simulink model "Model"  (R2024b)
settings: Solver=VariableStepAuto  StartTime=0.0  StopTime=30  MaxStep=0.001  RelTol=1e-4
PostLoadFcn:
  | SIM_setup
values from neighbouring files (symbols this model uses):
  A = 1.1    [RT14e_Parameters.m]    (also in RT15e_Parameters.m = 1.088; RT15evo_Parameters.m = 1.088; SIM_setup.m = 1.12)
  Aero_balance = 55    [RT14e_Parameters.m]    (also in RT15e_Parameters.m; RT15evo_Parameters.m; SIM_setup.m = 0.55)
  air_density = 1.29    [SIM_setup.m]
  Br_coef_of_friction_F = 0.33    [RT14e_Parameters.m]    (also in RT15e_Parameters.m; RT15evo_Parameters.m; SIM_setup.m = 0.25)
  Br_coef_of_friction_R = 0.33    [RT14e_Parameters.m]    (also in RT15e_Parameters.m; RT15evo_Parameters.m; SIM_setup.m = 0.25)
  Br_pistons_area_F = 3617.26/1e6    (= 0.00361726)    [RT14e_Parameters.m]    (also in RT15e_Parameters.m; RT15evo_Parameters.m; SIM_setup.m)
  Br_pistons_area_R = 2026.83/1e6    (= 0.00202683)    [RT14e_Parameters.m]    (also in RT15e_Parameters.m; RT15evo_Parameters.m; SIM_setup.m)
  Cd = 1.387    [SIM_setup.m]
  Cl = 3.299    [SIM_setup.m]
  CoG_z = 0.35    [RT14e_Parameters.m]    (also in RT15e_Parameters.m = 0.28495; RT15evo_Parameters.m = 0.28495; SIM_setup.m = 0.328)
  Default_Fz_F = g*(Mass*(Lr/Wheelbase))    [RT14e_Parameters.m]    (also in RT15e_Parameters.m; RT15evo_Parameters.m; SIM_setup.m = 608.22)
  Default_Fz_R = g*(Mass*(Lf/Wheelbase))    [RT14e_Parameters.m]    (also in RT15e_Parameters.m; RT15evo_Parameters.m; SIM_setup.m = 774.99)
  Effective_br_disk_r_F = 0.0905    [RT14e_Parameters.m]    (also in RT15e_Parameters.m; RT15evo_Parameters.m; SIM_setup.m)
  Effective_br_disk_r_R = 0.0895    [RT14e_Parameters.m]    (also in RT15e_Parameters.m; RT15evo_Parameters.m; SIM_setup.m)
  Fx = Data_Fx(2:end,3:end)    [RT14e_Parameters.m]    (also in RT15e_Parameters.m; RT15evo_Parameters.m; SIM_setup.m = Data_Fx(2:end,2:end))
  Fy = Data_Fy(2:end,3:end)    [RT14e_Parameters.m]    (also in RT15e_Parameters.m; RT15evo_Parameters.m; SIM_setup.m = Data_Fy(2:end,2:end))
  Fz = Data_Fy(2:end,2)    [RT14e_Parameters.m]    (also in RT15e_Parameters.m; RT15evo_Parameters.m; SIM_setup.m = Data_Fy(2:end,1))
  Half_track = 0.6    [SIM_setup.m]
  Iz_wehicle = 120    [RT14e_Parameters.m]    (also in RT15e_Parameters.m; RT15evo_Parameters.m; SIM_setup.m)
  Iz_wheel = 0.15    [RT14e_Parameters.m]    (also in RT15e_Parameters.m; RT15evo_Parameters.m; SIM_setup.m)
  Lateral_load_transfer_distribution = 0.55    [SIM_setup.m]
  Lf = Wheelbase - CoG_x    (= 0.77)    [RT14e_Parameters.m]    (also in RT15e_Parameters.m = 0.7504; RT15evo_Parameters.m = 0.7504; SIM_setup.m)
  Lr = Wheelbase - Lf    (= 0.755)    [RT14e_Parameters.m]    (also in RT15e_Parameters.m = 0.7746; RT15evo_Parameters.m = 0.7746; SIM_setup.m)
  Mass = Vehicle_mass + Driver_mass    (= 290)    [RT14e_Parameters.m]    (also in RT15e_Parameters.m = 265; RT15evo_Parameters.m; SIM_setup.m = 300)
  Max_Torque = 29.1    [SIM_setup.m]
  RB_torque_setting_1 = -2    [RT14e_Parameters.m]    (also in RT15e_Parameters.m; RT15evo_Parameters.m; SIM_setup.m)
  RB_torque_setting_10 = -20    [RT14e_Parameters.m]    (also in RT15e_Parameters.m; RT15evo_Parameters.m; SIM_setup.m)
  RB_torque_setting_2 = -4    [RT14e_Parameters.m]    (also in RT15e_Parameters.m; RT15evo_Parameters.m; SIM_setup.m)
  RB_torque_setting_3 = -6    [RT14e_Parameters.m]    (also in RT15e_Parameters.m; RT15evo_Parameters.m; SIM_setup.m)
  RB_torque_setting_4 = -8    [RT14e_Parameters.m]    (also in RT15e_Parameters.m; RT15evo_Parameters.m; SIM_setup.m)
  RB_torque_setting_5 = -10    [RT14e_Parameters.m]    (also in RT15e_Parameters.m; RT15evo_Parameters.m; SIM_setup.m)
  RB_torque_setting_6 = -12    [RT14e_Parameters.m]    (also in RT15e_Parameters.m; RT15evo_Parameters.m; SIM_setup.m)
  RB_torque_setting_7 = -14    [RT14e_Parameters.m]    (also in RT15e_Parameters.m; RT15evo_Parameters.m; SIM_setup.m)
  RB_torque_setting_8 = -16    [RT14e_Parameters.m]    (also in RT15e_Parameters.m; RT15evo_Parameters.m; SIM_setup.m)
  RB_torque_setting_9 = -18    [RT14e_Parameters.m]    (also in RT15e_Parameters.m; RT15evo_Parameters.m; SIM_setup.m)
  SA = Data_Fy(1,3:end)    [RT14e_Parameters.m]    (also in RT15e_Parameters.m; RT15evo_Parameters.m; SIM_setup.m = Data_Fy(1,2:end))
  SR = Data_Fx(1,3:end)    [RT14e_Parameters.m]    (also in RT15e_Parameters.m; RT15evo_Parameters.m; SIM_setup.m = Data_Fx(1,2:end))
  start_time = 182    [SIM_setup.m]
  start_velocity = Xsens_MTI_670_vel.Value(find(Xsens_MTI_670_vel.Time > start_time, 1)) * 1000 / 3600    [SIM_setup.m]
  Steering_angle_table = [0 9.9 19.9 30.14 40.57 51.05 61.29 70.87 79.38 91.9]    [SIM_setup.m]
  Steering_ratio_table = [3.25 3.24 3.23 3.20 3.16 3.10 3.04 2.97 2.90 2.77]    [SIM_setup.m]
  Tire_radius = 0.203    [RT14e_Parameters.m]    (also in RT15e_Parameters.m; RT15evo_Parameters.m; SIM_setup.m)
  Torque_limit_2 = Motor_maximum_torque*0.2    (= 5.82)    [RT14e_Parameters.m]    (also in RT15e_Parameters.m; RT15evo_Parameters.m; SIM_setup.m)
  Torque_limit_3 = Motor_maximum_torque*0.3    (= 8.73)    [RT14e_Parameters.m]    (also in RT15e_Parameters.m; RT15evo_Parameters.m; SIM_setup.m)
  Torque_limit_4 = Motor_maximum_torque*0.4    (= 11.64)    [RT14e_Parameters.m]    (also in RT15e_Parameters.m; RT15evo_Parameters.m; SIM_setup.m)
  Torque_limit_5 = Motor_maximum_torque*0.5    (= 14.55)    [RT14e_Parameters.m]    (also in RT15e_Parameters.m; RT15evo_Parameters.m; SIM_setup.m)
  Torque_limit_6 = Motor_maximum_torque*0.6    (= 17.46)    [RT14e_Parameters.m]    (also in RT15e_Parameters.m; RT15evo_Parameters.m; SIM_setup.m)
  Torque_limit_7 = Motor_maximum_torque*0.7    (= 20.37)    [RT14e_Parameters.m]    (also in RT15e_Parameters.m; RT15evo_Parameters.m; SIM_setup.m)
  Torque_limit_8 = Motor_maximum_torque*0.8    (= 23.28)    [RT14e_Parameters.m]    (also in RT15e_Parameters.m; RT15evo_Parameters.m; SIM_setup.m)
  Torque_limit_9 = 29.1    [RT14e_Parameters.m]    (also in RT15e_Parameters.m; RT15evo_Parameters.m; SIM_setup.m)
  Torque_limit_max = Motor_maximum_torque    (= 29.1)    [RT14e_Parameters.m]    (also in RT15e_Parameters.m; RT15evo_Parameters.m; SIM_setup.m)
  Torque_limit_min = Motor_maximum_torque*0.1    (= 2.91)    [RT14e_Parameters.m]    (also in RT15e_Parameters.m; RT15evo_Parameters.m; SIM_setup.m)
  Transmission_gear_ratio = 12.9    [SIM_setup.m]
  TV_RB_understeer_gradient_1 = -0.5    [RT14e_Parameters.m]    (also in RT15e_Parameters.m; RT15evo_Parameters.m; SIM_setup.m)
  TV_RB_understeer_gradient_10 = 0.005    [RT14e_Parameters.m]    (also in RT15e_Parameters.m; RT15evo_Parameters.m; SIM_setup.m)
  TV_RB_understeer_gradient_2 = -0.1    [RT14e_Parameters.m]    (also in RT15e_Parameters.m; RT15evo_Parameters.m; SIM_setup.m)
  TV_RB_understeer_gradient_3 = 0.08    [RT14e_Parameters.m]    (also in RT15e_Parameters.m; RT15evo_Parameters.m; SIM_setup.m)
  TV_RB_understeer_gradient_4 = 0.06    [RT14e_Parameters.m]    (also in RT15e_Parameters.m; RT15evo_Parameters.m; SIM_setup.m)
  TV_RB_understeer_gradient_5 = 0.05    [RT14e_Parameters.m]    (also in RT15e_Parameters.m; RT15evo_Parameters.m; SIM_setup.m)
  TV_RB_understeer_gradient_6 = 0.04    [RT14e_Parameters.m]    (also in RT15e_Parameters.m; RT15evo_Parameters.m; SIM_setup.m)
  TV_RB_understeer_gradient_7 = 0.03    [RT14e_Parameters.m]    (also in RT15e_Parameters.m; RT15evo_Parameters.m; SIM_setup.m)
  TV_RB_understeer_gradient_8 = 0.02    [RT14e_Parameters.m]    (also in RT15e_Parameters.m; RT15evo_Parameters.m; SIM_setup.m)
  TV_RB_understeer_gradient_9 = 0.01    [RT14e_Parameters.m]    (also in RT15e_Parameters.m; RT15evo_Parameters.m; SIM_setup.m)
  TV_understeer_gradient_1 = -0.5    [RT14e_Parameters.m]    (also in RT15e_Parameters.m; RT15evo_Parameters.m; SIM_setup.m)
  TV_understeer_gradient_10 = 0.002    [RT14e_Parameters.m]    (also in RT15e_Parameters.m; RT15evo_Parameters.m; SIM_setup.m)
  TV_understeer_gradient_2 = -0.1    [RT14e_Parameters.m]    (also in RT15e_Parameters.m; RT15evo_Parameters.m; SIM_setup.m)
  TV_understeer_gradient_3 = 0.06    [RT14e_Parameters.m]    (also in RT15e_Parameters.m; RT15evo_Parameters.m; SIM_setup.m)
  TV_understeer_gradient_4 = 0.05    [RT14e_Parameters.m]    (also in RT15e_Parameters.m; RT15evo_Parameters.m; SIM_setup.m)
  TV_understeer_gradient_5 = 0.04    [RT14e_Parameters.m]    (also in RT15e_Parameters.m; RT15evo_Parameters.m; SIM_setup.m)
  TV_understeer_gradient_6 = 0.03    [RT14e_Parameters.m]    (also in RT15e_Parameters.m; RT15evo_Parameters.m; SIM_setup.m)
  TV_understeer_gradient_7 = 0.02    [RT14e_Parameters.m]    (also in RT15e_Parameters.m; RT15evo_Parameters.m; SIM_setup.m)
  TV_understeer_gradient_8 = 0.01    [RT14e_Parameters.m]    (also in RT15e_Parameters.m; RT15evo_Parameters.m; SIM_setup.m)
  TV_understeer_gradient_9 = 0.005    [RT14e_Parameters.m]    (also in RT15e_Parameters.m; RT15evo_Parameters.m; SIM_setup.m)
  Wheel_base = 1.525    [SIM_setup.m]
  Wheel_rolling_resistance = 0.055    [RT14e_Parameters.m]    (also in RT15e_Parameters.m; RT15evo_Parameters.m; SIM_setup.m)
undefined symbols (not defined in the file or in its folder): Actual_Torque_Value_RL, Actual_Torque_Value_RR, aero_balance, APPS, Brake_Pressure_Front, Brake_Pressure_Rear, lateral_load_transfer_distribution, Steering_position, tire_radius, wheel_base, Xsens_MTI_670_accX, Xsens_MTI_670_accY, Xsens_MTI_670_gyrZ, Xsens_MTI_670_vel, Xsens_Yaw_Rate__deg_s_
libraries: simulink x20, simulink_extras x7, dspstat3 x4, slpidlib x1, slrealtimeloglib x1
(part 1 of 4)
settings Model: Creator=mordw  LastModifiedBy=RafałWarda(272419)
settings SolverCC: ZeroCrossAlgorithm=Adaptive
settings OptimizationCC: ReuseModelBlockBuffer=off
settings DebuggingCC: MaskedZcDiagnostic=none  IgnoredZcDiagnostic=none
settings RTWCC: GPUComputeCapability=3.5

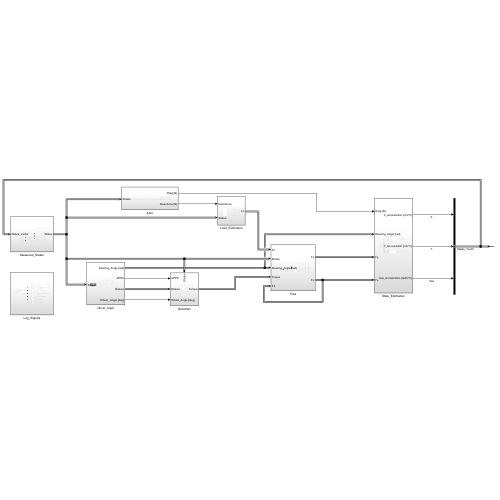
[thumbnail: Simulink's stored preview of the top-level diagram]
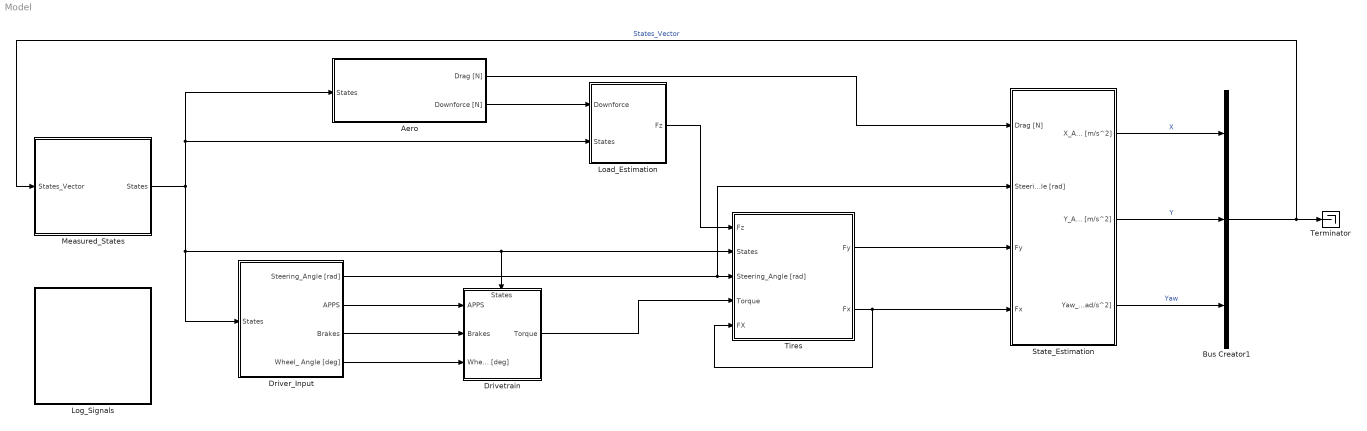
== system Model ==
  Aero : Subsystem
  Bus Creator1 : BusCreator  Inputs=3
  Driver_Input : Subsystem
  Drivetrain : Subsystem
      settings: PortSchema="{\"entries\":[{\"content\":{\"sides\":[{\"content\":{\"connectorIds\":[\"In1\",\"In2\",\"In3\"]},\"type\":\"ConnectorPlacement.EquallySpacedRectSide\",\"uuid\":\"ad6ef30a-e6d1-48a2-80ac-ce90815fbdb8\"},{\"content\":{\"connectorIds\":[\"Out1\"],\"side\":\"RIGHT\"},\"type\":\"ConnectorPlacement.EquallySpacedRectSide\",\"uuid\":\"754bb9ac-707b-4a43-9d55-0a5c68ba2719\"},{\"content\":{\"connectorIds\":[\"In4\"],\"side\":\"TOP\"},\"type\":\"ConnectorPlacement.EquallySpacedRectSide\",\"uuid\":\"92fbe14f-2b1b-4dfe-94da-640250e3fad1\"},{\"content\":{\"side\":\"BOTTOM\"},\"type\":\"ConnectorPlacement.EquallySpacedRectSide\",\"uuid\":\"78fbf731-d1bf-4d6d-863b-c8414bea3a73\"}]},\"type\":\"ConnectorPlacement.EquallySpacedConnector\",\"uuid\":\"eef32279-33f0-4d53-a445-a6b028ddce16\"}],\"packageUris\":[\"http://schema.mathworks.com/mf0/Connector/R2020b\"],\"version\":\"1.0\"}"
  Load_Estimation : Subsystem
  Log_Signals : Subsystem
  Measured_States : Subsystem
  State_Estimation : Subsystem
  Terminator : Terminator
  "Tires " : Subsystem
  wires:
  Driver_Input/1(Steering_Angle [rad]) -> State_Estimation/2(Steering_Angle [rad]), "Tires "/3(Steering_Angle [rad])
  Driver_Input/2(APPS) -> Drivetrain/1(APPS)
  Driver_Input/3(Brakes) -> Drivetrain/2(Brakes)
  State_Estimation/1(X_Acceleration [m/s^2]) -> Bus Creator1/1  "X"
  State_Estimation/2(Y_Acceleration [m/s^2]) -> Bus Creator1/2  "Y"
  State_Estimation/3(Yaw_Acceleration [rad/s^2]) -> Bus Creator1/3  "Yaw"
  Bus Creator1/1 -> Measured_States/1(States_Vector), Terminator/1  "States_Vector"
  Measured_States/1(States) -> Driver_Input/1(States), "Tires "/2(States), Drivetrain/4(States), Load_Estimation/2(States), Aero/1(States)
  Aero/1(Drag [N]) -> State_Estimation/1(Drag [N])
  Aero/2(Downforce [N]) -> Load_Estimation/1(Downforce)
  Load_Estimation/1(Fz) -> "Tires "/1(Fz)
  "Tires "/2(Fx) -> "Tires "/5(FX), State_Estimation/4(Fx)
  "Tires "/1(Fy) -> State_Estimation/3(Fy)
  Driver_Input/4(Wheel_ Angle [deg]) -> Drivetrain/3(Wheel_Angle [deg])
  Drivetrain/1(Torque) -> "Tires "/4(Torque)

== system Model/Aero ==
  States : Inport
  Bus Selector : BusSelector  OutputSignals=X/Y_Velocity [m/s].V_x [m/s]
  Gain1 : Gain  Gain=air_density
  Gain2 : Gain  Gain=1/2
  Gain3 : Gain  Gain=Cl
  Gain4 : Gain  Gain=A
  Gain5 : Gain  Gain=Cd
  Square : Math  Operator=square
  Drag [N] : Outport
  Downforce [N] : Outport  Port=2
  wires:
  Gain4/1 -> Gain1/1
  Gain3/1 -> Downforce [N]/1  "Downforce [N]"
  Gain1/1 -> Gain2/1
  Gain2/1 -> Gain5/1, Gain3/1
  Gain5/1 -> Drag [N]/1  "Drag [N]"
  Square/1 -> Gain4/1
  States/1 -> Bus Selector/1
  Bus Selector/1 -> Square/1  "<V_x [m/s]>"

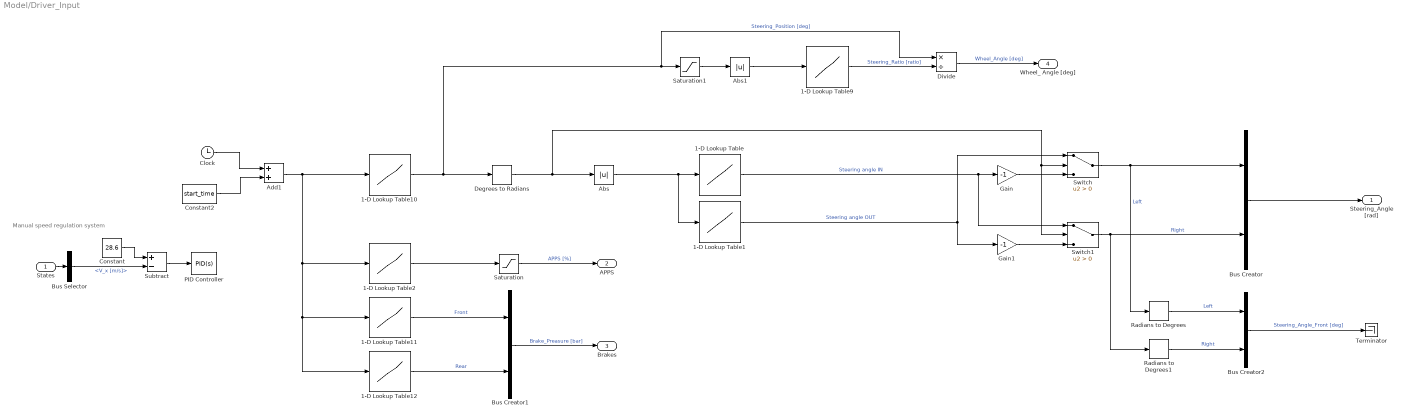
== system Model/Driver_Input ==
  note: Manual speed regulation system
  States : Inport
  1-D Lookup Table : Lookup_n-D  NumberOfTableDimensions=1  BreakpointsForDimension1=|  Table=|  InternalRulePriority=Speed  RndMeth=Simplest
      BreakpointsForDimension1=|
      | [0
      | 0.073230598
      | 0.146461196
      | 0.219691794
      | 0.292922392
      | 0.36615299
      | 0.439383588
      | 0.512614186
      | 0.585844784
      | 0.659075382
      | 0.73230598
      | 0.805536578
      | 0.878767176
      | 0.951997774
      | 1.025228372
      | 1.09845897
      | 1.171689568
      | 1.244920166
      | 1.318150764
      | 1.391381362
      | 1.46461196
      | 1.83076495]
      Table=|
      | [-0.000176278
      | 0.017065829
      | 0.034393458
      | 0.051818825
      | 0.069340186
      | 0.086971502
      | 0.104711028
      | 0.122574473
      | 0.140560091
      | 0.158685336
      | 0.176950206
      | 0.195370411
      | 0.21394595
      | 0.232697768
      | 0.251624118
      | 0.270745946
      | 0.290068486
      | 0.309609192
      | 0.3293733
      | 0.349386991
      | 0.369653754
      | 0.475541135]
  1-D Lookup Table1 : Lookup_n-D  NumberOfTableDimensions=1  BreakpointsForDimension1=|  Table=|  InternalRulePriority=Speed  RndMeth=Simplest
      BreakpointsForDimension1=|
      | [0
      | 0.073230598
      | 0.146461196
      | 0.219691794
      | 0.292922392
      | 0.36615299
      | 0.439383588
      | 0.512614186
      | 0.585844784
      | 0.659075382
      | 0.73230598
      | 0.805536578
      | 0.878767176
      | 0.951997774
      | 1.025228372
      | 1.09845897
      | 1.171689568
      | 1.244920166
      | 1.318150764
      | 1.391381362
      | 1.46461196
      | 1.83076495]
      Table=|
      | [0.000176278
      | 0.017336355
      | 0.034421384
      | 0.051433108
      | 0.068382
      | 0.085266315
      | 0.102098271
      | 0.118877866
      | 0.135613828
      | 0.152304412
      | 0.168961834
      | 0.18558435
      | 0.202182431
      | 0.218754332
      | 0.235310526
      | 0.251851011
      | 0.26838277
      | 0.284907547
      | 0.301432324
      | 0.317960592
      | 0.334499332
      | 0.417475776]
  1-D Lookup Table10 : Lookup_n-D  NumberOfTableDimensions=1  BreakpointsForDimension1=Steering_position.Time  Table=Steering_position.Value  InternalRulePriority=Speed  RndMeth=Simplest
  1-D Lookup Table11 : Lookup_n-D  NumberOfTableDimensions=1  BreakpointsForDimension1=Brake_Pressure_Front.Time  Table=Brake_Pressure_Front.Value  InternalRulePriority=Speed  RndMeth=Simplest
  1-D Lookup Table12 : Lookup_n-D  NumberOfTableDimensions=1  BreakpointsForDimension1=Brake_Pressure_Rear.Time  Table=Brake_Pressure_Rear.Value  InternalRulePriority=Speed  RndMeth=Simplest
  1-D Lookup Table2 : Lookup_n-D  NumberOfTableDimensions=1  BreakpointsForDimension1=APPS.Time  Table=APPS.Value  InternalRulePriority=Speed  RndMeth=Simplest
  1-D Lookup Table9 : Lookup_n-D  NumberOfTableDimensions=1  BreakpointsForDimension1=Steering_angle_table  Table=Steering_ratio_table  InternalRulePriority=Speed  RndMeth=Simplest
  Abs : Abs  SaturateOnIntegerOverflow=off
  Abs1 : Abs  SaturateOnIntegerOverflow=off
  Add1 : Sum
  Bus Creator : BusCreator  Inputs=2
  Bus Creator1 : BusCreator  Inputs=2
  Bus Creator2 : BusCreator  Inputs=2
  Bus Selector : BusSelector  OutputSignals=X/Y_Velocity [m/s].V_x [m/s]
  Clock : Clock
  Constant : Constant  Value=28.6
  Constant2 : Constant  Value=start_time
  Degrees to Radians : simulink_extras/Transformations/Degrees to Radians
  Divide : Product  Inputs=*/
  Gain : Gain  Gain=-1
  Gain1 : Gain  Gain=-1
  PID Controller : slpidlib/PID Controller  Controller=PID  Form=Parallel  TimeDomain=Continuous-time  UseExternalTs=off  SampleTime=-1  IntegratorMethod=Forward Euler  FilterMethod=Forward Euler  ControllerParametersSource=internal  P=50  I=20  UseKiTs=off  D=0  UseExternalDerivativeSource=off  N=100  UseFilter=on  TunerSelectOption=Transfer Function Based (PID Tuner App)  InitialConditionSource=internal  InitialConditionForIntegrator=0  InitialConditionForFilter=0  DifferentiatorICPrevScaledInput=0  ExternalReset=none  TrackingMode=off  Kt=1  LimitOutput=off  SatLimitsSource=internal  UpperSaturationLimit=inf  LowerSaturationLimit=-inf  LinearizeAsGain=on  AntiWindupMode=none  Kb=1  LimitIntegrator=off  UpperIntegratorSaturationLimit=inf  LowerIntegratorSaturationLimit=-inf  POutMin=[]  POutMax=[]  IOutMin=[]  IOutMax=[]  DOutMin=[]  DOutMax=[]  NOutMin=[]  NOutMax=[]  SumOutMin=[]  SumOutMax=[]  SaturationOutMin=[]  SaturationOutMax=[]  PParamMin=[]  PParamMax=[]  IParamMin=[]  IParamMax=[]  DParamMin=[]  DParamMax=[]  NParamMin=[]  NParamMax=[]  KbParamMin=[]  KbParamMax=[]  KtParamMin=[]  KtParamMax=[]  KbOutMin=[]  KbOutMax=[]  KtOutMin=[]  KtOutMax=[]  IntegratorOutMin=[]  IntegratorOutMax=[]  FilterOutMin=[]  FilterOutMax=[]  SumI1OutMin=[]  SumI1OutMax=[]  SumI2OutMin=[]  SumI2OutMax=[]  SumI3OutMin=[]  SumI3OutMax=[]  SumI4OutMin=[]  SumI4OutMax=[]  SumDOutMin=[]  SumDOutMax=[]  DifferentiatorOutMin=[]  DifferentiatorOutMax=[]  FilterDiffOutCoefMin=[]  FilterDiffOutCoefMax=[]  ReciprocalOutMin=[]  ReciprocalOutMax=[]  SumDenOutMin=[]  SumDenOutMax=[]  SumNumOutMin=[]  SumNumOutMax=[]  DivideOutMin=[]  DivideOutMax=[]  UdiffTsProdOutMin=[]  UdiffTsProdOutMax=[]  NTsProdOutMin=[]  NTsProdOutMax=[]  UintegralTsProdOutMin=[]  UintegralTsProdOutMax=[]  UngainTsProdOutMin=[]  UngainTsProdOutMax=[]  ClampingZeroOutDataTypeStr=Inherit: Inherit via back propagation  ClampingZeroOutMin=[]  ClampingZeroOutMax=[]  FilterDenConstantOutDataTypeStr=Inherit: Inherit via back propagation  FilterDenConstantOutMin=[]  FilterDenConstantOutMax=[]  PCopyOutDataTypeStr=Inherit: Inherit via back propagation  PCopyOutMin=[]  PCopyOutMax=[]  NCopyOutDataTypeStr=Inherit: Inherit via back propagation  NCopyOutMin=[]  NCopyOutMax=[]  IntegratorContinuousStateAttributes=''  IntegratorStateMustResolveToSignalObject=off  IntegratorRTWStateStorageClass=Auto  FilterContinuousStateAttributes=''  FilterStateMustResolveToSignalObject=off  FilterRTWStateStorageClass=Auto  ParallelPVariant=InternalParameters  IdealPVariant=Disabled  IVariant=InternalParameters  DVariant=InternalParameters  IntegratorVariant=Continuous  SatVariant=Disabled  AWVariant=Passthrough  PCopyVariant=Disabled  TRVariant=Disabled  FdbkBlocksVariant=Forward  IdealPFdbkVariant=Disabled  SatFdbkVariant=Disabled  DerivativeFilterVariant=ContFilter  NVariant=InternalParameters  NCopyVariant=Disabled  FilterICVariant=InternalICsFilter  IntegratorICVariant=InternalICs  ExternalResetVariant=Disabled  TRSumVariant=Passthrough  SumFdbkVariant=Disabled  SumVariant=Sum_PID  TsampFilterVariant=InternalTs  TsampNgainVariant=Passthrough  TsampIntegralVariant=Disabled_SignalSpec  ExternalSaturationOutDataTypeStr=Inherit: Same as second input  DerivativeSourceVariant=ErrorSignal  PreIntVariant=InternalPreInt
  Radians to Degrees : simulink_extras/Transformations/Radians to Degrees
  Radians to Degrees1 : simulink_extras/Transformations/Radians to Degrees
  Saturation : Saturate  UpperLimit=100  LowerLimit=0
  Saturation1 : Saturate  UpperLimit=110  LowerLimit=-110
  Subtract : Sum  Inputs=+-
  Switch : Switch  Criteria=u2 > Threshold  SaturateOnIntegerOverflow=off  InputSameDT=off
  Switch1 : Switch  Criteria=u2 > Threshold  SaturateOnIntegerOverflow=off  InputSameDT=off
  Terminator : Terminator
  Steering_Angle [rad] : Outport
  APPS : Outport  Port=2
  Brakes : Outport  Port=3
  Wheel_ Angle [deg] : Outport  Port=4
  wires:
  1-D Lookup Table1/1 -> Gain1/1, Switch/1  "Steering angle OUT"
  1-D Lookup Table/1 -> Gain/1, Switch1/1  "Steering angle IN"
  Radians to Degrees1/1 -> Bus Creator2/2  "Right"
  Radians to Degrees/1 -> Bus Creator2/1  "Left"
  Bus Creator/1 -> Steering_Angle [rad]/1
  Switch1/1 -> Bus Creator/2, Radians to Degrees1/1  "Right"
  Switch/1 -> Bus Creator/1, Radians to Degrees/1  "Left"
  Saturation/1 -> APPS/1  "APPS [%]"
  Abs/1 -> 1-D Lookup Table1/1, 1-D Lookup Table/1
  Degrees to Radians/1 -> Switch/2, Switch1/2, Abs/1
  Gain/1 -> Switch/3
  Gain1/1 -> Switch1/3
  Clock/1 -> Add1/1
  Bus Creator1/1 -> Brakes/1  "Brake_Preasure [bar]"
  Divide/1 -> Wheel_ Angle [deg]/1  "Wheel_Angle [deg]"
  1-D Lookup Table9/1 -> Divide/2  "Steering_Ratio [ratio]"
  Saturation1/1 -> Abs1/1
  Abs1/1 -> 1-D Lookup Table9/1
  1-D Lookup Table10/1 -> Divide/1, Saturation1/1, Degrees to Radians/1  "Steering_Position [deg]"
  1-D Lookup Table11/1 -> Bus Creator1/1  "Front"
  1-D Lookup Table12/1 -> Bus Creator1/2  "Rear"
  Constant2/1 -> Add1/2
  Add1/1 -> 1-D Lookup Table12/1, 1-D Lookup Table11/1, 1-D Lookup Table2/1, 1-D Lookup Table10/1
  1-D Lookup Table2/1 -> Saturation/1
  Bus Creator2/1 -> Terminator/1  "Steering_Angle_Front [deg]"
  Bus Selector/1 -> Subtract/2  "<V_x [m/s]>"
  Subtract/1 -> PID Controller/1
  Constant/1 -> Subtract/1
  States/1 -> Bus Selector/1

== system Model/Drivetrain ==
  APPS : Inport
  Brakes : Inport  Port=2
  Wheel_Angle [deg] : Inport  Port=3
  States : Inport  Port=4
  1-D Lookup Table : Lookup_n-D  NumberOfTableDimensions=1  BreakpointsForDimension1=[0 100]  Table=[0 29.1]  InternalRulePriority=Speed  RndMeth=Simplest
  Braking_Torque : Subsystem
  Bus Creator1 : BusCreator  Inputs=2
  Bus Creator : BusCreator  Inputs=2
  Engine_Power : Subsystem
  Gain1 : Gain  Gain=Transmission_gear_ratio
  Gain2 : Gain  Gain=Transmission_gear_ratio
  TV Algorithm : Subsystem  Commented=on
      settings: PortSchema="{\"entries\":[{\"content\":{\"sides\":[{\"content\":{\"connectorIds\":[\"In1\",\"In2\"]},\"type\":\"ConnectorPlacement.EquallySpacedRectSide\",\"uuid\":\"7b07616b-0ebd-48b3-9298-597f7dd07d66\"},{\"content\":{\"connectorIds\":[\"Out1\",\"Out2\"],\"side\":\"RIGHT\"},\"type\":\"ConnectorPlacement.EquallySpacedRectSide\",\"uuid\":\"1ca9a803-29a7-4f66-83a1-4b3325ff94c2\"},{\"content\":{\"connectorIds\":[\"In3\",\"In4\"],\"side\":\"TOP\"},\"type\":\"ConnectorPlacement.EquallySpacedRectSide\",\"uuid\":\"ce1bec80-9762-4372-b362-27bcbf1a4c54\"}]},\"type\":\"ConnectorPlacement.EquallySpacedConnector\",\"uuid\":\"fe6232db-ec4c-42e2-b838-1cb40525fabf\"}],\"packageUris\":[\"http://schema.mathworks.com/mf0/Connector/R2020b\"],\"version\":\"1.0\"}"
  Terminator1 : Terminator
  Torque : Outport
  wires:
  Bus Creator/1 -> Torque/1
  APPS/1 -> 1-D Lookup Table/1
  Gain2/1 -> Bus Creator1/1  "Left"
  Gain1/1 -> Bus Creator1/2  "Right"
  Bus Creator1/1 -> Bus Creator/1, Engine_Power/1(Wheel_Torque)  "Wheel_Torque_Rear"
  Brakes/1 -> TV Algorithm/1(Brakes), Braking_Torque/1(Brake_Pressure [bar])  "Brake_Pressure [bar]"
  States/1 -> TV Algorithm/3(States)
  Wheel_Angle [deg]/1 -> TV Algorithm/4(Wheel Angle F [deg])
  1-D Lookup Table/1 -> Gain1/1, Gain2/1  "Motor_Torque"
  Engine_Power/1(Energy_Used_Per_Engine [kWh]) -> Terminator1/1  "Energy_Used_Per_Engine [kWh]"
  Braking_Torque/1(Brake_Torque [Nm]) -> Bus Creator/2  "Brake_Torque [Nm]"

== system Model/Load_Estimation ==
  Downforce : Inport
  States : Inport  Port=2
  Add{,1..3} (4 alike) : Sum  Inputs=+++
  Bus Creator : BusCreator  Inputs=4
  Constant1 : Constant  Value=Default_Fz_F
  Constant2 : Constant  Value=Default_Fz_R
  Constant3 : Constant  Value=Default_Fz_R
  Constant5 : Constant  Value=Default_Fz_F
  Gain : Gain  Gain=Aero_balance
  Gain1 : Gain  Gain=1/2
  Gain2 : Gain  Gain=1/2
  Load_Transfer : Subsystem
  Subtract : Sum  Inputs=+-
  Fz : Outport
  tag scope: Fz_RL=global, Fz_RR=global
  wires:
  Add3/1 -> [Fz_RR], Bus Creator/4  "Fz_RR"
  Add2/1 -> Bus Creator/3, [Fz_RL]  "Fz_RL"
  Add1/1 -> Bus Creator/2  "Fz_FR"
  Add/1 -> Bus Creator/1  "Fz_FL"
  Bus Creator/1 -> Fz/1  "Fz_Load [N]"
  States/1 -> Load_Transfer/1(In1)
  Constant5/1 -> Add/3  "Fz_FL"
  Constant1/1 -> Add1/3  "Fz_FR"
  Constant2/1 -> Add2/3  "Fz_RL"
  Constant3/1 -> Add3/3  "Fz_RR"
  Downforce/1 -> Gain/1, Subtract/1
  Gain/1 -> Gain2/1, Subtract/2  "Downforce_Rear"
  Subtract/1 -> Gain1/1
  Load_Transfer/1(FL) -> Add/1
  Load_Transfer/2(FR) -> Add1/1
  Load_Transfer/3(RL) -> Add2/1
  Load_Transfer/4(RR) -> Add3/1
  Gain1/1 -> Add/2, Add1/2
  Gain2/1 -> Add3/2, Add2/2

== system Model/Log_Signals ==
  1-D Lookup Table1 : Lookup_n-D  NumberOfTableDimensions=1  BreakpointsForDimension1=Actual_Torque_Value_RL.Time  Table=Actual_Torque_Value_RL.Value  InternalRulePriority=Speed  RndMeth=Simplest
  1-D Lookup Table2 : Lookup_n-D  NumberOfTableDimensions=1  BreakpointsForDimension1=Actual_Torque_Value_RR.Time  Table=Actual_Torque_Value_RR.Value  InternalRulePriority=Speed  RndMeth=Simplest
  1-D Lookup Table3 : Lookup_n-D  NumberOfTableDimensions=1  BreakpointsForDimension1=Xsens_MTI_670_accX.Time  Table=Xsens_MTI_670_accX.Value  InternalRulePriority=Speed  RndMeth=Simplest
  1-D Lookup Table4 : Lookup_n-D  NumberOfTableDimensions=1  BreakpointsForDimension1=Xsens_MTI_670_vel.Time  Table=Xsens_MTI_670_vel.Value  InternalRulePriority=Speed  RndMeth=Simplest
  1-D Lookup Table5 : Lookup_n-D  Commented=on  NumberOfTableDimensions=1  BreakpointsForDimension1=Xsens_Yaw_Rate__deg_s_.Time  Table=Xsens_Yaw_Rate__deg_s_.Value  InternalRulePriority=Speed  RndMeth=Simplest
  1-D Lookup Table6 : Lookup_n-D  NumberOfTableDimensions=1  BreakpointsForDimension1=Xsens_MTI_670_accY.Time  Table=Xsens_MTI_670_accY.Value  InternalRulePriority=Speed  RndMeth=Simplest
  1-D Lookup Table7 : Lookup_n-D  NumberOfTableDimensions=1  BreakpointsForDimension1=Xsens_MTI_670_gyrZ.Time  Table=Xsens_MTI_670_gyrZ.Value  InternalRulePriority=Speed  RndMeth=Simplest
  Add1 : Sum
  Clock : Clock
  Constant2 : Constant  Value=start_time
  Gain : Gain  Gain=1000/3600
  Gain1 : Gain  Gain=-1
  Gain4 : Gain  Gain=-1
  Moving Average : dspstat3/Moving Average  Method=Sliding window  ForgettingFactorPort=off  SpecifyWindowLength=on  WindowLength=50  OverlapLength=49  AllowArbitraryInputLength=off  ForgettingFactor=0.9  SimulateUsing=Code generation
  Moving Average1 : dspstat3/Moving Average  Method=Sliding window  ForgettingFactorPort=off  SpecifyWindowLength=on  WindowLength=50  OverlapLength=49  AllowArbitraryInputLength=off  ForgettingFactor=0.9  SimulateUsing=Code generation
  Radians to Degrees : simulink_extras/Transformations/Radians to Degrees
  Terminator{1,3..7} (6 alike) : Terminator
  Terminator2 : Terminator  Commented=on
  wires:
  1-D Lookup Table6/1 -> Moving Average/1
  1-D Lookup Table5/1 -> Terminator2/1  "Yaw_Rate_Log"
  1-D Lookup Table4/1 -> Gain/1  "X_Velocity_Log"
  Gain4/1 -> Terminator4/1  "Y_Acceleration_Log"
  Moving Average/1 -> Gain4/1
  Add1/1 -> 1-D Lookup Table5/1, 1-D Lookup Table7/1, 1-D Lookup Table2/1, 1-D Lookup Table1/1, 1-D Lookup Table4/1, 1-D Lookup Table3/1, 1-D Lookup Table6/1
  Clock/1 -> Add1/1
  Constant2/1 -> Add1/2
  1-D Lookup Table1/1 -> Terminator1/1  "Torque_RL_Log"
  1-D Lookup Table2/1 -> Terminator5/1  "Torque_RR_Log"
  1-D Lookup Table3/1 -> Moving Average1/1
  Moving Average1/1 -> Terminator6/1  "X_Acceleration_Log"
  Gain/1 -> Terminator3/1  "X_Velocity_Log"
  Radians to Degrees/1 -> Terminator7/1  "Yaw_Rate_Log"
  1-D Lookup Table7/1 -> Gain1/1
  Gain1/1 -> Radians to Degrees/1

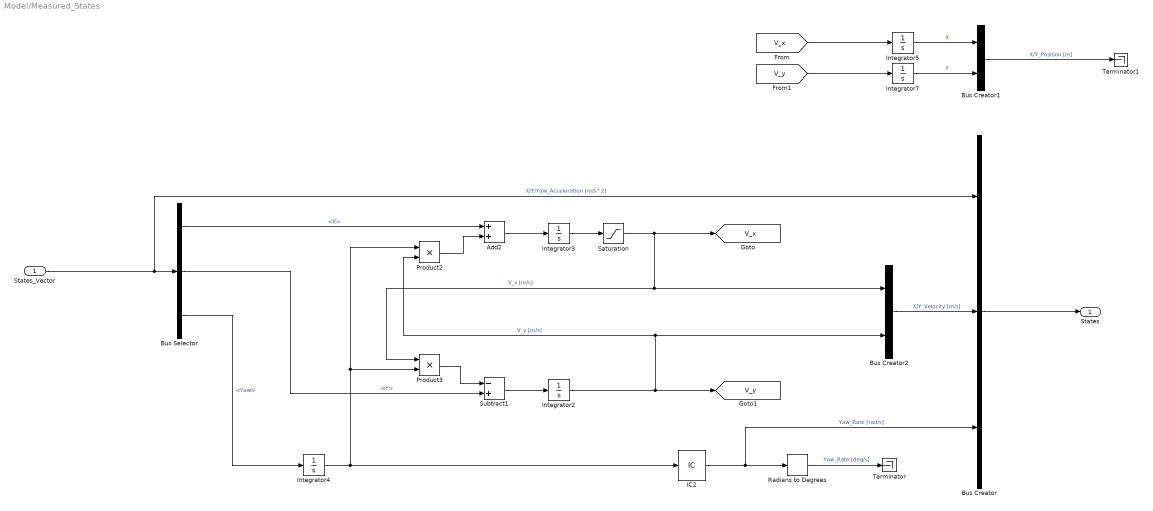
== system Model/Measured_States ==
  States_Vector : Inport
  Add2 : Sum
  Bus Creator : BusCreator  Inputs=3
  Bus Creator1 : BusCreator  Inputs=2
  Bus Creator2 : BusCreator  Inputs=V_x [m/s],V_y [m/s]
  Bus Selector : BusSelector  OutputSignals=X,Y,Yaw
  IC2 : InitialCondition
  Integrator{2,4..5,7} (4 alike) : Integrator
  Integrator3 : Integrator  InitialCondition=start_velocity
  Product2 : Product
  Product3 : Product
  Radians to Degrees : simulink_extras/Transformations/Radians to Degrees
  Saturation : Saturate  UpperLimit=inf  LowerLimit=0.5
  Subtract1 : Sum  Inputs=-+
  Terminator : Terminator
  Terminator1 : Terminator
  States : Outport
  tag scope: V_x=global, V_y=global
  wires:
  States_Vector/1 -> Bus Creator/1, Bus Selector/1  "X/Y/Yaw_Acceleration [m/s^2]"
  Bus Selector/1 -> Add2/1  "<X>"
  Bus Selector/2 -> Subtract1/2  "<Y>"
  Bus Selector/3 -> Integrator4/1  "<Yaw>"
  Integrator3/1 -> Saturation/1
  Bus Creator/1 -> States/1
  Radians to Degrees/1 -> Terminator/1  "Yaw_Rate [deg/s]"
  IC2/1 -> Bus Creator/3, Radians to Degrees/1  "Yaw_Rate [rad/s]"
  Integrator7/1 -> Bus Creator1/2  "Y"
  Integrator5/1 -> Bus Creator1/1  "X"
  Bus Creator1/1 -> Terminator1/1  "X/Y_Position [m]"
  Bus Creator2/1 -> Bus Creator/2  "X/Y_Velocity [m/s]"
  Integrator2/1 -> Product2/2, Bus Creator2/2, [V_y]  "V_y [m/s]"
  Product2/1 -> Add2/2
  Add2/1 -> Integrator3/1
  Integrator4/1 -> IC2/1, Product2/1, Product3/2
  Product3/1 -> Subtract1/1
  Saturation/1 -> Product3/1, Bus Creator2/1, [V_x]  "V_x [m/s]"
  Subtract1/1 -> Integrator2/1
  [V_x] -> Integrator5/1
  [V_y] -> Integrator7/1

== system Model/State_Estimation ==
  Drag [N] : Inport
  Steering_Angle [rad] : Inport  Port=2
  Fy : Inport  Port=3
  Fx : Inport  Port=4
  IC : InitialCondition  Value=0.1
  IC1 : InitialCondition  Value=0.1
  IC2 : InitialCondition  Value=0.1
  Lateral_Acceleration : Subsystem
  Longitudinal_Acceleration : Subsystem
  Yaw_Acceleration : Subsystem
  X_Acceleration [m/s^2] : Outport
  Y_Acceleration [m/s^2] : Outport  Port=2
  Yaw_Acceleration [rad/s^2] : Outport  Port=3
  wires:
  Steering_Angle [rad]/1 -> Lateral_Acceleration/1(Steering_Angle [rad]), Longitudinal_Acceleration/2(Steering_Angle [rad]), Yaw_Acceleration/1(Wheel_Angels [rad])
  Fx/1 -> Lateral_Acceleration/2(Fx [N]), Longitudinal_Acceleration/3(Fx), Yaw_Acceleration/2(X_Tire_Forces [N])
  Fy/1 -> Lateral_Acceleration/3(Fy [N]), Longitudinal_Acceleration/4(Fy), Yaw_Acceleration/3(Y_Tire_Forces [N])
  Drag [N]/1 -> Longitudinal_Acceleration/1(Drag [N])
  Yaw_Acceleration/1(Yaw_Acceleration [rad/s^2]) -> IC/1
  IC2/1 -> X_Acceleration [m/s^2]/1
  IC/1 -> Yaw_Acceleration [rad/s^2]/1
  IC1/1 -> Y_Acceleration [m/s^2]/1
  Longitudinal_Acceleration/1(X_Acceleration [m/s^2]) -> IC2/1
  Lateral_Acceleration/1(Y_Acceleration [m/s^2]) -> IC1/1

== system Model/Tires  ==
  Fz : Inport
  States : Inport  Port=2
  Steering_Angle [rad] : Inport  Port=3
  Torque : Inport  Port=4
  FX : Inport  Port=5
  Bus Creator3 : BusCreator  Inputs=3
  Bus Creator4 : BusCreator  Inputs=4
  Bus Creator5 : BusCreator  Inputs=4
  Bus Selector : BusSelector  OutputSignals=X/Y_Velocity [m/s].V_x [m/s],X/Y_Velocity [m/s].V_y [m/s],Yaw_Rate [rad/s]
  FL : Subsystem
  FR : Subsystem
  RL : Subsystem
  RR : Subsystem
  Subsystem1 : Subsystem
      settings: PortSchema="{\"entries\":[{\"content\":{\"sides\":[{\"content\":{\"connectorIds\":[\"In1\",\"In2\",\"In3\",\"In4\",\"In5\",\"In6\"]},\"type\":\"ConnectorPlacement.EquallySpacedRectSide\",\"uuid\":\"4c3e8c63-25c2-4cb7-8078-3e31b06e7546\"},{\"content\":{\"connectorIds\":[\"Out1\",\"Out2\"],\"side\":\"RIGHT\"},\"type\":\"ConnectorPlacement.EquallySpacedRectSide\",\"uuid\":\"1572fde6-1871-4f20-824d-3c71aef7d818\"},{\"content\":{\"side\":\"TOP\"},\"type\":\"ConnectorPlacement.EquallySpacedRectSide\",\"uuid\":\"71d93f94-a5a8-4ca6-8e92-c4c9a50b1024\"},{\"content\":{\"connectorIds\":[\"In7\"],\"side\":\"BOTTOM\"},\"type\":\"ConnectorPlacement.EquallySpacedRectSide\",\"uuid\":\"c0e5b51d-0cfd-4c37-9571-746b70176797\"}]},\"type\":\"ConnectorPlacement.EquallySpacedConnector\",\"uuid\":\"bf3ccf88-c513-41f7-aec5-380bb57a5870\"}],\"packageUris\":[\"http://schema.mathworks.com/mf0/Connector/R2020b\"],\"version\":\"1.0\"}"
  Fy : Outport
  Fx : Outport  Port=2
  wires:
  Torque/1 -> Subsystem1/1(Torque)
  FX/1 -> Subsystem1/2(Fx)
  Bus Selector/3 -> Subsystem1/5(Yaw_Rate [rad/s])  "<Yaw_Rate [rad/s]>"
  Subsystem1/1(Slip_Ratio) -> Bus Creator3/1  "Slip_Ratio"
  Subsystem1/2(Slip_Angle [deg]) -> Bus Creator3/2  "Slip_Angle [deg]"
  Bus Creator3/1 -> FL/1(In1), FR/1(In1), RR/1(In1), RL/1(In1)
  FL/1(Fx_FL) -> Bus Creator4/1  "FL"
  FR/1(Fx_FR) -> Bus Creator4/2  "FR"
  RL/1(Fx_RL) -> Bus Creator4/3  "RL"
  RR/1(Fx_RR) -> Bus Creator4/4  "RR"
  FL/2(Fy_FL) -> Bus Creator5/1  "FL"
  FR/2(Fy_FR) -> Bus Creator5/2  "FR"
  RL/2(Fy_RL) -> Bus Creator5/3  "RL"
  RR/2(Fy_RR) -> Bus Creator5/4  "RR"
  Bus Creator4/1 -> Fx/1  "Fx_Wheels [N]"
  Bus Creator5/1 -> Fy/1  "Fy_Wheels [N]"
  States/1 -> Bus Selector/1
  Fz/1 -> Subsystem1/7(Fz), Bus Creator3/3  "Fz"
  Steering_Angle [rad]/1 -> Subsystem1/6(Steering_Angle [rad])
  Bus Selector/2 -> Subsystem1/4(Y_Velocity [m/s])  "<V_y [m/s]>"
  Bus Selector/1 -> Subsystem1/3(X_Velocity [m/s])  "<V_x [m/s]>"

== system Model/Drivetrain/Braking_Torque ==
  Brake_Pressure [bar] : Inport
  Braking_Torque_Front : Subsystem
  Braking_Torque_Rear : Subsystem
  Bus Creator : BusCreator  Inputs=2
  Bus Creator1 : BusCreator  Inputs=2
  Bus Creator2 : BusCreator  Inputs=2
  Bus Selector : BusSelector  OutputSignals=Front,Rear
  Gain{,1..3} (4 alike) : Gain  Gain=0.5
  Brake_Torque [Nm] : Outport
  wires:
  Bus Selector/2 -> Braking_Torque_Rear/1(Brake_Pressure [bar])  "<Rear>"
  Bus Creator2/1 -> Brake_Torque [Nm]/1  "Brake_Torque [Nm]"
  Braking_Torque_Front/1(Braking torque [Nm]) -> Gain/1, Gain1/1
  Bus Selector/1 -> Braking_Torque_Front/1(Brake_Pressure [bar])  "<Front>"
  Brake_Pressure [bar]/1 -> Bus Selector/1
  Bus Creator/1 -> Bus Creator2/1  "Front"
  Gain/1 -> Bus Creator/1  "FR"
  Gain1/1 -> Bus Creator/2  "FL"
  Gain3/1 -> Bus Creator1/2  "RL"
  Braking_Torque_Rear/1(Braking_Torque [Nm]) -> Gain2/1, Gain3/1
  Bus Creator1/1 -> Bus Creator2/2  "Rear"
  Gain2/1 -> Bus Creator1/1  "RR"

== system Model/Drivetrain/Engine_Power ==
  Wheel_Torque : Inport
  Bus Creator : BusCreator  Inputs=2
  Bus Selector : BusSelector  OutputSignals=RL,RR
  Bus Selector1 : BusSelector  OutputSignals=Left,Right
  Engine_RL : Subsystem
  Engine_RR : Subsystem
  Energy_Used_Per_Engine [kWh] : Outport
  wires:
  [WAS] -> Bus Selector/1
  Bus Selector/1 -> Engine_RL/1(Wheel_Angular_Speed)  "<RL>"
  Bus Selector/2 -> Engine_RR/1(Wheel_Angular_Speed)  "<RR>"
  Wheel_Torque/1 -> Bus Selector1/1
  Bus Selector1/1 -> Engine_RL/2(Engine_Torque)  "<Left>"
  Bus Selector1/2 -> Engine_RR/2(Engine_Torque)  "<Right>"
  Engine_RL/1(Energy Used [kWh]) -> Bus Creator/1  "Energy_Used_Engine_RL [kWh]"
  Engine_RR/1(Energy Used [kWh]) -> Bus Creator/2  "Energy_Used_Engine_RR [kWh]"
  Bus Creator/1 -> Energy_Used_Per_Engine [kWh]/1  "Energy_Used_Per_Engine [kWh]"

== system Model/Drivetrain/TV Algorithm ==
  Brakes : Inport
  Positive Torque Command [Nm] : Inport  Port=2
  States : Inport  Port=3
  Wheel Angle F [deg] : Inport  Port=4
  Bus Selector : BusSelector  OutputSignals=Yaw_Rate [rad/s],Y,X,V_x [m/s],V_y [m/s]
  Radians to Degrees : simulink_extras/Transformations/Radians to Degrees
  Subsystem : Subsystem
  Torque Vectoring : Subsystem
  Commanded Torque RL [Nm] : Outport
  Commanded Torque RR [Nm] : Outport  Port=2
  wires:
  States/1 -> Bus Selector/1
  Bus Selector/1 -> Radians to Degrees/1  "<Yaw_Rate [rad/s]>"
  Torque Vectoring/1(Torque After TV RL [Nm]) -> Commanded Torque RL [Nm]/1  "Torque After TV RL [Nm]"
  Torque Vectoring/2(Torque After TV RR [Nm]) -> Commanded Torque RR [Nm]/1  "Torque After TV RL [Nm]"
  Wheel Angle F [deg]/1 -> Torque Vectoring/8(Wheel Angle F [deg])
  Bus Selector/2 -> Torque Vectoring/5(Xsens accY [m/s2])  "<Y>"
  Bus Selector/3 -> Torque Vectoring/6(Xsens accX [m/s2])  "<X>"
  Bus Selector/4 -> Torque Vectoring/9(Vehicle Speed [km/h])  "<V_x [m/s]>"
  Positive Torque Command [Nm]/1 -> Torque Vectoring/2(Positive Torque Command RR [Nm]), Torque Vectoring/1(Positive Torque Command RL [Nm])
  Brakes/1 -> Torque Vectoring/7(Brakes)

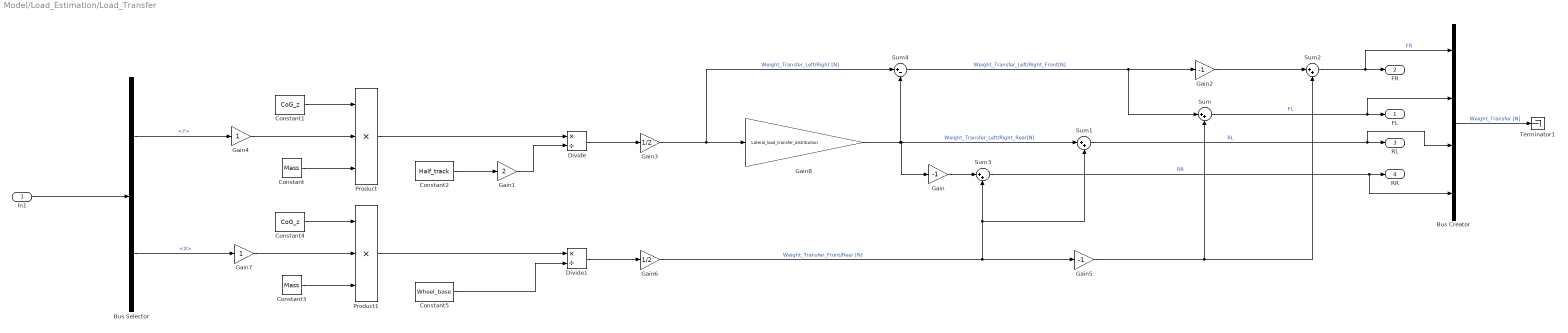
== system Model/Load_Estimation/Load_Transfer ==
  In1 : Inport
  Bus Creator : BusCreator  Inputs=4
  Bus Selector : BusSelector  OutputSignals=X/Y/Yaw_Acceleration [m/s^2].Y,X/Y/Yaw_Acceleration [m/s^2].X
  Constant : Constant  Value=Mass
  Constant1 : Constant  Value=CoG_z
  Constant2 : Constant  Value=Half_track
  Constant3 : Constant  Value=Mass
  Constant4 : Constant  Value=CoG_z
  Constant5 : Constant  Value=Wheel_base
  Divide : Product  Inputs=*/
  Divide1 : Product  Inputs=*/
  Gain : Gain  Gain=-1
  Gain1 : Gain  Gain=2
  Gain2 : Gain  Gain=-1
  Gain3 : Gain  Gain=1/2
  Gain4 : Gain
  Gain5 : Gain  Gain=-1
  Gain6 : Gain  Gain=1/2
  Gain7 : Gain
  Gain8 : Gain  Gain=Lateral_load_transfer_distribution
  Product : Product  Inputs=3
  Product1 : Product  Inputs=3
  Sum{,1..3} (4 alike) : Sum  Inputs=|++
  Sum4 : Sum  Inputs=|+-
  Terminator1 : Terminator
  FL : Outport
  FR : Outport  Port=2
  RL : Outport  Port=3
  RR : Outport  Port=4
  wires:
  In1/1 -> Bus Selector/1
  Bus Selector/1 -> Gain4/1  "<Y>"
  Constant/1 -> Product/3
  Constant1/1 -> Product/1
  Product/1 -> Divide/1
  Constant2/1 -> Gain1/1
  Divide/1 -> Gain3/1
  Gain1/1 -> Divide/2
  Gain4/1 -> Product/2
  Gain7/1 -> Product1/2
  Constant5/1 -> Divide1/2
  Divide1/1 -> Gain6/1
  Product1/1 -> Divide1/1
  Constant4/1 -> Product1/1
  Constant3/1 -> Product1/3
  Bus Selector/2 -> Gain7/1  "<X>"
  Gain6/1 -> Gain5/1, Sum1/2, Sum3/2  "Weight_Transfer_Front/Rear [N]"
  Sum/1 -> Bus Creator/2, FL/1  "FL"
  Sum1/1 -> Bus Creator/3, RL/1  "RL"
  Sum2/1 -> Bus Creator/1, FR/1  "FR"
  Gain2/1 -> Sum2/1
  Sum3/1 -> Bus Creator/4, RR/1  "RR"
  Gain/1 -> Sum3/1
  Gain5/1 -> Sum2/2, Sum/2
  Gain3/1 -> Sum4/1, Gain8/1  "Weight_Transfer_Left/Right [N]"
  Gain8/1 -> Sum4/2, Sum1/1, Gain/1  "Weight_Transfer_Left/Right_Rear[N]"
  Sum4/1 -> Sum/1, Gain2/1  "Weight_Transfer_Left/Right_Front[N]"
  Bus Creator/1 -> Terminator1/1  "Weight_Transfer [N]"

== system Model/State_Estimation/Lateral_Acceleration ==
  Steering_Angle [rad] : Inport
  Fx [N] : Inport  Port=2
  Fy [N] : Inport  Port=3
  Add1 : Sum  Inputs=++++++
  Bus Selector : BusSelector  OutputSignals=FL,FR
  Bus Selector1 : BusSelector  OutputSignals=FL,FR,RL,RR
  Cos : Trigonometry  Operator=cos
  Cos1 : Trigonometry  Operator=cos
  Demux : Demux  Outputs=2
  Gain : Gain  Gain=1/Mass
  Product{,1..3} (4 alike) : Product
  Sin : Trigonometry
  Sin1 : Trigonometry
  Y_Acceleration [m/s^2] : Outport
  wires:
  Steering_Angle [rad]/1 -> Demux/1
  Fy [N]/1 -> Bus Selector1/1
  Fx [N]/1 -> Bus Selector/1
  Demux/1 -> Sin/1, Cos/1  "Steering_Angle_FL"
  Demux/2 -> Sin1/1, Cos1/1  "Steering_Angle_FR"
  Product/1 -> Add1/1
  Product1/1 -> Add1/2
  Product2/1 -> Add1/3
  Product3/1 -> Add1/4
  Bus Selector/2 -> Product3/2  "<FR>"
  Bus Selector/1 -> Product2/2  "<FL>"
  Sin/1 -> Product2/1
  Sin1/1 -> Product3/1
  Cos/1 -> Product/1
  Cos1/1 -> Product1/1
  Bus Selector1/1 -> Product/2  "<FL>"
  Bus Selector1/2 -> Product1/2  "<FR>"
  Bus Selector1/3 -> Add1/5  "<RL>"
  Bus Selector1/4 -> Add1/6  "<RR>"
  Add1/1 -> Gain/1  "Fy_Sum [N]"
  Gain/1 -> Y_Acceleration [m/s^2]/1

== system Model/State_Estimation/Longitudinal_Acceleration ==
  Drag [N] : Inport
  Steering_Angle [rad] : Inport  Port=2
  Fx : Inport  Port=3
  Fy : Inport  Port=4
  Add1 : Sum  Inputs=++++++-
  Bus Selector1 : BusSelector  OutputSignals=FL,FR
  Bus Selector2 : BusSelector  OutputSignals=FL,FR,RL,RR
  Cos : Trigonometry  Operator=cos
  Cos1 : Trigonometry  Operator=cos
  Demux : Demux  Outputs=2
  Gain1 : Gain  Gain=-1
  Gain2 : Gain  Gain=-1
  Gain3 : Gain  Gain=1/Mass
  Product{,1..3} (4 alike) : Product
  Sin : Trigonometry
  Sin1 : Trigonometry
  X_Acceleration [m/s^2] : Outport
  wires:
  Steering_Angle [rad]/1 -> Demux/1
  Demux/1 -> Cos/1, Gain1/1  "Steering_Angle_FL"
  Demux/2 -> Gain2/1, Cos1/1  "Steering_Angle_FR"
  Fx/1 -> Bus Selector2/1
  Gain1/1 -> Sin/1
  Gain2/1 -> Sin1/1
  Product/1 -> Add1/2
  Cos1/1 -> Product/1
  Cos/1 -> Product1/1
  Product1/1 -> Add1/1
  Product3/1 -> Add1/5
  Product2/1 -> Add1/6
  Drag [N]/1 -> Add1/7
  Fy/1 -> Bus Selector1/1
  Sin/1 -> Product3/1
  Bus Selector1/1 -> Product3/2  "<FL>"
  Bus Selector1/2 -> Product2/1  "<FR>"
  Bus Selector2/1 -> Product1/2  "<FL>"
  Bus Selector2/2 -> Product/2  "<FR>"
  Bus Selector2/3 -> Add1/3  "<RL>"
  Bus Selector2/4 -> Add1/4  "<RR>"
  Sin1/1 -> Product2/2
  Add1/1 -> Gain3/1  "Fx_Sum [N]"
  Gain3/1 -> X_Acceleration [m/s^2]/1

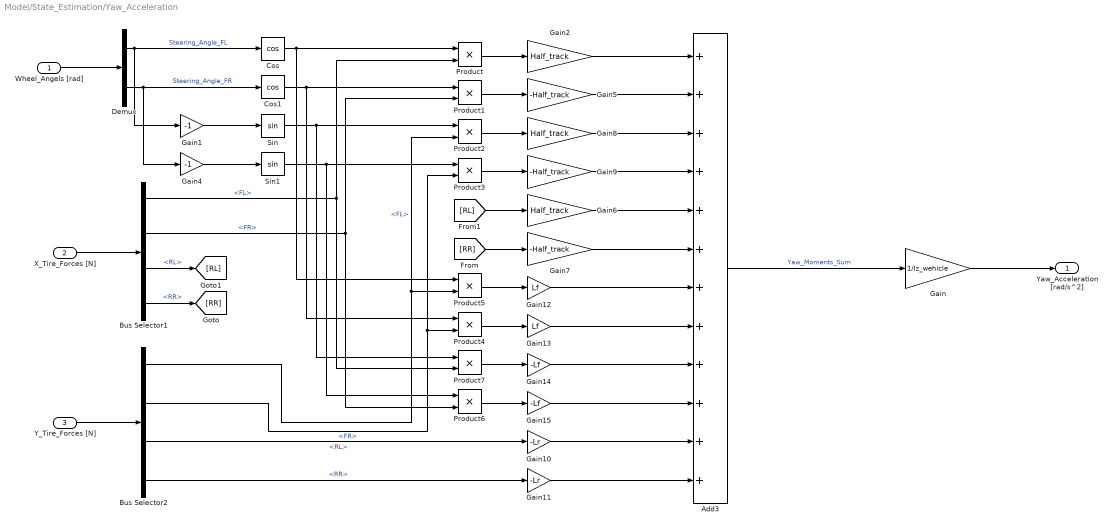
== system Model/State_Estimation/Yaw_Acceleration ==
  Wheel_Angels [rad] : Inport
  X_Tire_Forces [N] : Inport  Port=2
  Y_Tire_Forces [N] : Inport  Port=3
  Add3 : Sum  Inputs=++++++++++++
  Bus Selector1 : BusSelector  OutputSignals=FL,FR,RL,RR
  Bus Selector2 : BusSelector  OutputSignals=FL,FR,RL,RR
  Cos : Trigonometry  Operator=cos
  Cos1 : Trigonometry  Operator=cos
  Demux : Demux  Outputs=2
  Gain : Gain  Gain=1/Iz_wehicle
  Gain1 : Gain  Gain=-1
  Gain10 : Gain  Gain=-Lr
  Gain11 : Gain  Gain=-Lr
  Gain12 : Gain  Gain=Lf
  Gain13 : Gain  Gain=Lf
  Gain14 : Gain  Gain=-Lf
  Gain15 : Gain  Gain=-Lf
  Gain2 : Gain  Gain=Half_track
  Gain4 : Gain  Gain=-1
  Gain5 : Gain  Gain=-Half_track
  Gain6 : Gain  Gain=Half_track
  Gain7 : Gain  Gain=-Half_track
  Gain8 : Gain  Gain=Half_track
  Gain9 : Gain  Gain=-Half_track
  Product{,1..7} (8 alike) : Product
  Sin : Trigonometry
  Sin1 : Trigonometry
  Yaw_Acceleration [rad/s^2] : Outport
  wires:
  Add3/1 -> Gain/1  "Yaw_Moments_Sum"
  Gain/1 -> Yaw_Acceleration [rad/s^2]/1
  Gain4/1 -> Sin1/1
  Wheel_Angels [rad]/1 -> Demux/1
  Gain1/1 -> Sin/1
  Demux/1 -> Gain1/1, Cos/1  "Steering_Angle_FL"
  Demux/2 -> Cos1/1, Gain4/1  "Steering_Angle_FR"
  Y_Tire_Forces [N]/1 -> Bus Selector2/1
  Cos/1 -> Product/1, Product5/1
  Cos1/1 -> Product1/1, Product4/1
  Product/1 -> Gain2/1
  Product1/1 -> Gain5/1
  Sin/1 -> Product2/1, Product7/1
  Product2/1 -> Gain8/1
  Sin1/1 -> Product3/1, Product6/1
  Product5/1 -> Gain12/1
  Product4/1 -> Gain13/1
  Product6/1 -> Gain15/1
  Product7/1 -> Gain14/1
  X_Tire_Forces [N]/1 -> Bus Selector1/1
  Bus Selector1/2 -> Product6/2, Product1/2  "<FR>"
  Bus Selector1/1 -> Product/2, Product7/2  "<FL>"
  Bus Selector2/2 -> Product4/2, Product3/2  "<FR>"
  Bus Selector2/1 -> Product5/2, Product2/2  "<FL>"
  Gain2/1 -> Add3/1
  Gain5/1 -> Add3/2
  Gain6/1 -> Add3/5
  Gain7/1 -> Add3/6
  Gain8/1 -> Add3/3
  Gain9/1 -> Add3/4
  Product3/1 -> Gain9/1
  Bus Selector2/3 -> Gain10/1  "<RL>"
  Gain10/1 -> Add3/11
  Gain11/1 -> Add3/12
  Bus Selector2/4 -> Gain11/1  "<RR>"
  Gain12/1 -> Add3/7
  Gain13/1 -> Add3/8
  Gain14/1 -> Add3/9
  Gain15/1 -> Add3/10
  [RR] -> Gain7/1
  Bus Selector1/4 -> [RR]  "<RR>"
  [RL] -> Gain6/1
  Bus Selector1/3 -> [RL]  "<RL>"

== system Model/Tires /FL ==
  In1 : Inport
  2-D Lookup Table : Lookup_n-D  BreakpointsForDimension1=Fz  BreakpointsForDimension2=SA  Table=Fy  InternalRulePriority=Speed  RndMeth=Simplest
      settings: InputPortMap=u0,u1
  2-D Lookup Table1 : Lookup_n-D  BreakpointsForDimension1=Fz  BreakpointsForDimension2=SR  Table=Fx  InternalRulePriority=Speed  RndMeth=Simplest
      settings: InputPortMap=u0,u1
  Bus Selector : BusSelector  OutputSignals=Slip_Ratio.Slip_Ratio_FL,Fz.Fz_FL,Slip_Angle [deg].Slip_Angle_FL
  Fx_FL : Outport
  Fy_FL : Outport  Port=2
  wires:
  2-D Lookup Table/1 -> Fy_FL/1
  2-D Lookup Table1/1 -> Fx_FL/1
  Bus Selector/1 -> 2-D Lookup Table1/2  "<Slip_Ratio_FL>"
  In1/1 -> Bus Selector/1
  Bus Selector/3 -> 2-D Lookup Table/2  "<Slip_Angle_FL>"
  Bus Selector/2 -> 2-D Lookup Table/1, 2-D Lookup Table1/1  "<Fz_FL>"

== system Model/Tires /FR ==
  In1 : Inport
  2-D Lookup Table : Lookup_n-D  BreakpointsForDimension1=Fz  BreakpointsForDimension2=SA  Table=Fy  InternalRulePriority=Speed  RndMeth=Simplest
      settings: InputPortMap=u0,u1
  2-D Lookup Table1 : Lookup_n-D  BreakpointsForDimension1=Fz  BreakpointsForDimension2=SR  Table=Fx  InternalRulePriority=Speed  RndMeth=Simplest
      settings: InputPortMap=u0,u1
  Bus Selector : BusSelector  OutputSignals=Slip_Ratio.Slip_Ratio_FR,Fz.Fz_FR,Slip_Angle [deg].Slip_Angle_FR
  Fx_FR : Outport
  Fy_FR : Outport  Port=2
  wires:
  2-D Lookup Table1/1 -> Fx_FR/1
  2-D Lookup Table/1 -> Fy_FR/1
  In1/1 -> Bus Selector/1
  Bus Selector/1 -> 2-D Lookup Table1/2  "<Slip_Ratio_FR>"
  Bus Selector/3 -> 2-D Lookup Table/2  "<Slip_Angle_FR>"
  Bus Selector/2 -> 2-D Lookup Table/1, 2-D Lookup Table1/1  "<Fz_FR>"

== system Model/Tires /RL ==
  In1 : Inport
  2-D Lookup Table : Lookup_n-D  BreakpointsForDimension1=Fz  BreakpointsForDimension2=SA  Table=Fy  InternalRulePriority=Speed  RndMeth=Simplest
      settings: InputPortMap=u0,u1
  2-D Lookup Table1 : Lookup_n-D  BreakpointsForDimension1=Fz  BreakpointsForDimension2=SR  Table=Fx  InternalRulePriority=Speed  RndMeth=Simplest
      settings: InputPortMap=u0,u1
  Bus Selector : BusSelector  OutputSignals=Slip_Ratio.Slip_Ratio_RL,Fz.Fz_RL,Slip_Angle [deg].Slip_Angle_RL
  Fx_RL : Outport
  Fy_RL : Outport  Port=2
  wires:
  2-D Lookup Table/1 -> Fy_RL/1
  In1/1 -> Bus Selector/1
  Bus Selector/1 -> 2-D Lookup Table1/2  "<Slip_Ratio_RL>"
  Bus Selector/3 -> 2-D Lookup Table/2  "<Slip_Angle_RL>"
  Bus Selector/2 -> 2-D Lookup Table1/1, 2-D Lookup Table/1  "<Fz_RL>"
  2-D Lookup Table1/1 -> Fx_RL/1

== system Model/Tires /RR ==
  In1 : Inport
  2-D Lookup Table : Lookup_n-D  BreakpointsForDimension1=Fz  BreakpointsForDimension2=SA  Table=Fy  InternalRulePriority=Speed  RndMeth=Simplest
      settings: InputPortMap=u0,u1
  2-D Lookup Table1 : Lookup_n-D  BreakpointsForDimension1=Fz  BreakpointsForDimension2=SR  Table=Fx  InternalRulePriority=Speed  RndMeth=Simplest
      settings: InputPortMap=u0,u1
  Bus Selector : BusSelector  OutputSignals=Slip_Ratio.Slip_Ratio_RR,Fz.Fz_RR,Slip_Angle [deg].Slip_Angle_RR
  Fx_RR : Outport
  Fy_RR : Outport  Port=2
  wires:
  In1/1 -> Bus Selector/1
  2-D Lookup Table/1 -> Fy_RR/1
  Bus Selector/1 -> 2-D Lookup Table1/2  "<Slip_Ratio_RR>"
  Bus Selector/3 -> 2-D Lookup Table/2  "<Slip_Angle_RR>"
  Bus Selector/2 -> 2-D Lookup Table/1, 2-D Lookup Table1/1  "<Fz_RR>"
  2-D Lookup Table1/1 -> Fx_RR/1

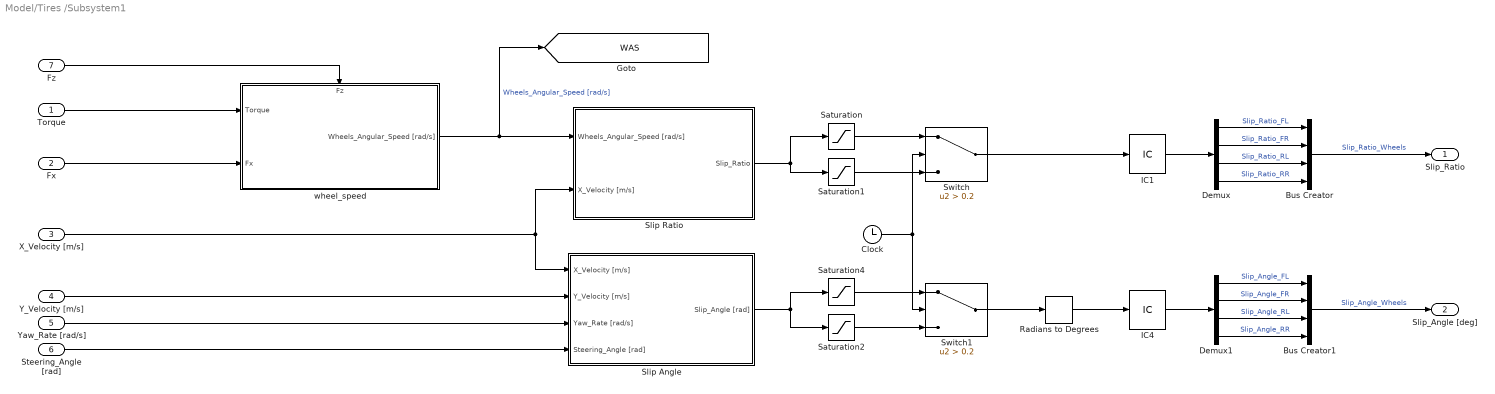
== system Model/Tires /Subsystem1 ==
  Torque : Inport
  Fx : Inport  Port=2
  X_Velocity [m/s] : Inport  Port=3
  Y_Velocity [m/s] : Inport  Port=4
  Yaw_Rate [rad/s] : Inport  Port=5
  Steering_Angle [rad] : Inport  Port=6
  Fz : Inport  Port=7
  Bus Creator : BusCreator  Inputs=4
  Bus Creator1 : BusCreator  Inputs=4
  Clock : Clock
  Demux : Demux
  Demux1 : Demux
  IC1 : InitialCondition  Value=0
  IC4 : InitialCondition  Value=0
  Radians to Degrees : simulink_extras/Transformations/Radians to Degrees
  Saturation : Saturate  UpperLimit=0.2  LowerLimit=-0.2
  Saturation1 : Saturate  UpperLimit=0.05  LowerLimit=-0.05
  Saturation2 : Saturate  UpperLimit=0.01  LowerLimit=-0.01
  Saturation4 : Saturate  UpperLimit=0.35  LowerLimit=-0.35
  Slip Angle : Subsystem
  Slip Ratio : Subsystem
  Switch : Switch  Criteria=u2 > Threshold  Threshold=0.2  SaturateOnIntegerOverflow=off  InputSameDT=off
  Switch1 : Switch  Criteria=u2 > Threshold  Threshold=0.2  SaturateOnIntegerOverflow=off  InputSameDT=off
  wheel_speed : Subsystem
      settings: PortSchema="{\"entries\":[{\"content\":{\"sides\":[{\"content\":{\"connectorIds\":[\"In1\",\"In2\"]},\"type\":\"ConnectorPlacement.EquallySpacedRectSide\",\"uuid\":\"15092166-14ce-458f-8814-c8c529b404ff\"},{\"content\":{\"connectorIds\":[\"Out1\"],\"side\":\"RIGHT\"},\"type\":\"ConnectorPlacement.EquallySpacedRectSide\",\"uuid\":\"66225d7f-0835-4a54-ba48-dd0fc21c3b18\"},{\"content\":{\"connectorIds\":[\"In3\"],\"side\":\"TOP\"},\"type\":\"ConnectorPlacement.EquallySpacedRectSide\",\"uuid\":\"e640b56a-2f04-4291-8d41-f01328ba15b5\"}]},\"type\":\"ConnectorPlacement.EquallySpacedConnector\",\"uuid\":\"87946f02-b44c-4e08-9031-15e47f027ea8\"}],\"packageUris\":[\"http://schema.mathworks.com/mf0/Connector/R2020b\"],\"version\":\"1.0\"}"
  Slip_Ratio : Outport
  Slip_Angle [deg] : Outport  Port=2
  tag scope: WAS=global
  wires:
  wheel_speed/1(Wheels_Angular_Speed [rad/s]) -> [WAS], Slip Ratio/1(Wheels_Angular_Speed [rad/s])  "Wheels_Angular_Speed [rad/s]"
  X_Velocity [m/s]/1 -> Slip Ratio/2(X_Velocity [m/s]), Slip Angle/1(X_Velocity [m/s])
  Slip Ratio/1(Slip_Ratio) -> Saturation/1, Saturation1/1
  Torque/1 -> wheel_speed/1(Torque)
  Radians to Degrees/1 -> IC4/1
  Y_Velocity [m/s]/1 -> Slip Angle/2(Y_Velocity [m/s])
  Slip Angle/1(Slip_Angle [rad]) -> Saturation2/1, Saturation4/1
  Steering_Angle [rad]/1 -> Slip Angle/4(Steering_Angle [rad])
  Fx/1 -> wheel_speed/2(Fx)
  Yaw_Rate [rad/s]/1 -> Slip Angle/3(Yaw_Rate [rad/s])
  Demux/1 -> Bus Creator/1  "Slip_Ratio_FL"
  Demux/2 -> Bus Creator/2  "Slip_Ratio_FR"
  Demux/3 -> Bus Creator/3  "Slip_Ratio_RL"
  Demux/4 -> Bus Creator/4  "Slip_Ratio_RR"
  Bus Creator/1 -> Slip_Ratio/1  "Slip_Ratio_Wheels"
  Demux1/4 -> Bus Creator1/4  "Slip_Angle_RR"
  Demux1/3 -> Bus Creator1/3  "Slip_Angle_RL"
  Demux1/2 -> Bus Creator1/2  "Slip_Angle_FR"
  Demux1/1 -> Bus Creator1/1  "Slip_Angle_FL"
  IC4/1 -> Demux1/1
  Bus Creator1/1 -> Slip_Angle [deg]/1  "Slip_Angle_Wheels"
  Saturation/1 -> Switch/1
  Saturation1/1 -> Switch/3
  Saturation4/1 -> Switch1/1
  Saturation2/1 -> Switch1/3
  Fz/1 -> wheel_speed/3(Fz)
  Switch1/1 -> Radians to Degrees/1
  Switch/1 -> IC1/1
  IC1/1 -> Demux/1
  Clock/1 -> Switch/2, Switch1/2
